simulink model "RailP_PRV"  (R2016b)
settings: configuration reference "CodeGenConfigSet" (kept outside this file)
values from neighbouring files (symbols this model uses):
  PRV_ClosePressureMin_C = Calibration.Parameter    [init_RailP_PRV.m]
  PRV_ctOpnMax_C = Calibration.Parameter    [init_RailP_PRV.m]
  PRV_dpRPGradOpn_CA0 = Calibration.Parameter    [init_RailP_PRV.m]
  PRV_dpRPGradOpn_CA1 = Calibration.Parameter    [init_RailP_PRV.m]
  PRV_nClsdMax_C = Calibration.Parameter    [init_RailP_PRV.m]
  PRV_nMinPresInc_C = Calibration.Parameter    [init_RailP_PRV.m]
  PRV_nOpnMin_C = Calibration.Parameter    [init_RailP_PRV.m]
  PRV_pAvrgRPTol_C = Calibration.Parameter    [init_RailP_PRV.m]
  PRV_tiCalcAvrgRP_C = Calibration.Parameter    [init_RailP_PRV.m]
  PRV_tiOpnMax_C = Calibration.Parameter    [init_RailP_PRV.m]
  PRV_tiWaitAvrgRP_C = Calibration.Parameter    [init_RailP_PRV.m]
  PRV_tiWaitNVld_C = Calibration.Parameter    [init_RailP_PRV.m]
  PRV_tiWaitPresInc_C = Calibration.Parameter    [init_RailP_PRV.m]
undefined symbols (not defined in the file or in its folder): PRV_State_conv, RailP_PRV_DT
settings Model: Creator=liutao  LastModifiedBy=shiliwei
settings ConfigSetRef: SourceLocation=Base Workspace

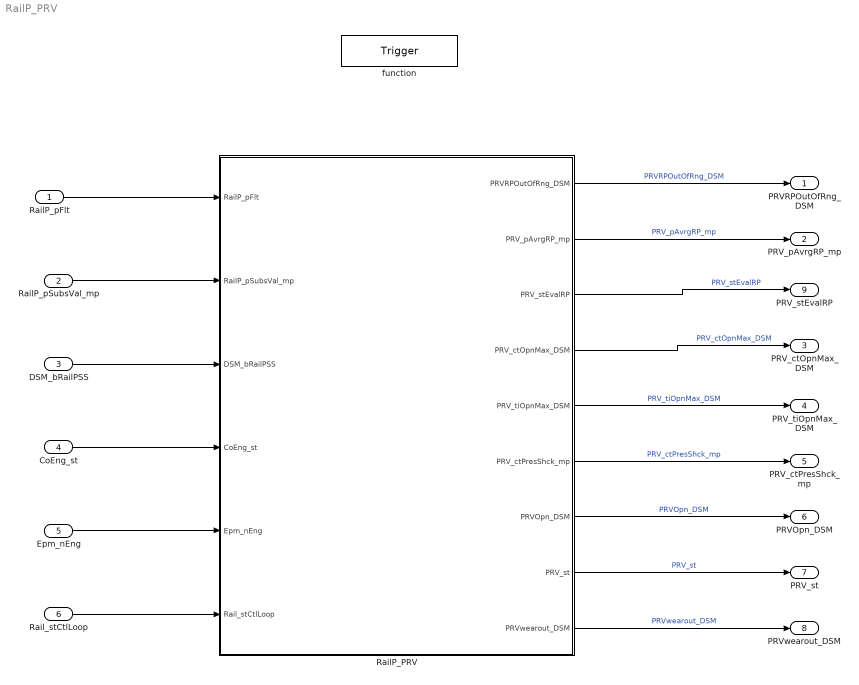
== system RailP_PRV ==
  RailP_pFlt : Inport  Tag=bar  Description=Maximum rail pressure of the last 10 sampling cycle  OutMin=0  OutMax=2500  OutDataTypeStr=RailPressure_bar
  RailP_pSubsVal_mp : Inport  Tag=bar  Description=Rail pressure substitution value in case of an error in pressure sensor  Port=2  OutMin=0  OutMax=2500  OutDataTypeStr=RailPressure_bar
  DSM_bRailPSS : Inport  Description=Status of FId_RailPSS  Port=3  OutMin=0  OutMax=1  OutDataTypeStr=boolean
  CoEng_st : Inport  Description=Engine coordinator state  Port=4  OutDataTypeStr=Enum: EngState_conv
  Epm_nEng : Inport  Tag=rpm  Description=Engine speed  Port=5  OutMin=0  OutMax=6000  OutDataTypeStr=EngSpeed_rpm
  Rail_stCtlLoop : Inport  Description=State of the rail pressure governor control  Port=6  OutDataTypeStr=Enum: RailCtl_State_conv
  function : TriggerPort  TriggerType=function-call  VariantControl=Variant
  RailP_PRV : Subsystem  TreatAsAtomicUnit=on
  PRVRPOutOfRng_DSM : Outport  Description=Averaged rail pressure is outside the expected tolerance range  OutMin=0  OutMax=1  OutDataTypeStr=boolean
  PRV_pAvrgRP_mp : Outport  Tag=bar  Description=|  Port=2  OutMin=0  OutMax=2000  OutDataTypeStr=RailPressure_bar
      | averaged rail pressure for detection of an opened
      | pressure relief valve by the rail pressure evaluation
  PRV_ctOpnMax_DSM : Outport  Description=Maximum number of opening cycles till wear out of PRV  Port=3  OutMin=0  OutMax=1  OutDataTypeStr=boolean
  PRV_tiOpnMax_DSM : Outport  Description=Maximum open time till wear out of PRV  Port=4  OutMin=0  OutMax=1  OutDataTypeStr=boolean
  PRV_ctPresShck_mp : Outport  Description=|  Port=5  OutMin=0  OutMax=6000  OutDataTypeStr=State_uint16
      | number of performed rail pressure shock cycles to
      | force the opening of the pressure relief valve
  PRVOpn_DSM : Outport  Description=PRV valve open state diagnostic  Port=6  OutMin=0  OutMax=1  OutDataTypeStr=boolean
  PRV_st : Outport  Description=state variable of the pressure relief valve  Port=7  OutDataTypeStr=Enum: PRV_State_conv
  PRVwearout_DSM : Outport  Description=PRV valve open counters or duration beyond setpoint value  Port=8  OutMin=0  OutMax=1  OutDataTypeStr=boolean
  PRV_stEvalRP : Outport  Description=state variable of the rail pressure evaluation for the recognition of the opening of the pressure relief valve  Port=9  OutDataTypeStr=Enum: PRV_EVALRPState_conv
  wires:
  RailP_PRV/1(PRVRPOutOfRng_DSM) -> PRVRPOutOfRng_DSM/1  "PRVRPOutOfRng_DSM"
  RailP_PRV/2(PRV_pAvrgRP_mp) -> PRV_pAvrgRP_mp/1  "PRV_pAvrgRP_mp"
  RailP_PRV/4(PRV_ctOpnMax_DSM) -> PRV_ctOpnMax_DSM/1  "PRV_ctOpnMax_DSM"
  RailP_PRV/5(PRV_tiOpnMax_DSM) -> PRV_tiOpnMax_DSM/1  "PRV_tiOpnMax_DSM"
  RailP_PRV/6(PRV_ctPresShck_mp) -> PRV_ctPresShck_mp/1  "PRV_ctPresShck_mp"
  RailP_PRV/7(PRVOpn_DSM) -> PRVOpn_DSM/1  "PRVOpn_DSM"
  RailP_PRV/8(PRV_st) -> PRV_st/1  "PRV_st"
  RailP_PRV/9(PRVwearout_DSM) -> PRVwearout_DSM/1  "PRVwearout_DSM"
  RailP_pFlt/1 -> RailP_PRV/1(RailP_pFlt)
  RailP_pSubsVal_mp/1 -> RailP_PRV/2(RailP_pSubsVal_mp)
  Rail_stCtlLoop/1 -> RailP_PRV/6(Rail_stCtlLoop)
  Epm_nEng/1 -> RailP_PRV/5(Epm_nEng)
  CoEng_st/1 -> RailP_PRV/4(CoEng_st)
  DSM_bRailPSS/1 -> RailP_PRV/3(DSM_bRailPSS)
  RailP_PRV/3("PRV_stEvalRP ") -> PRV_stEvalRP/1  "PRV_stEvalRP"

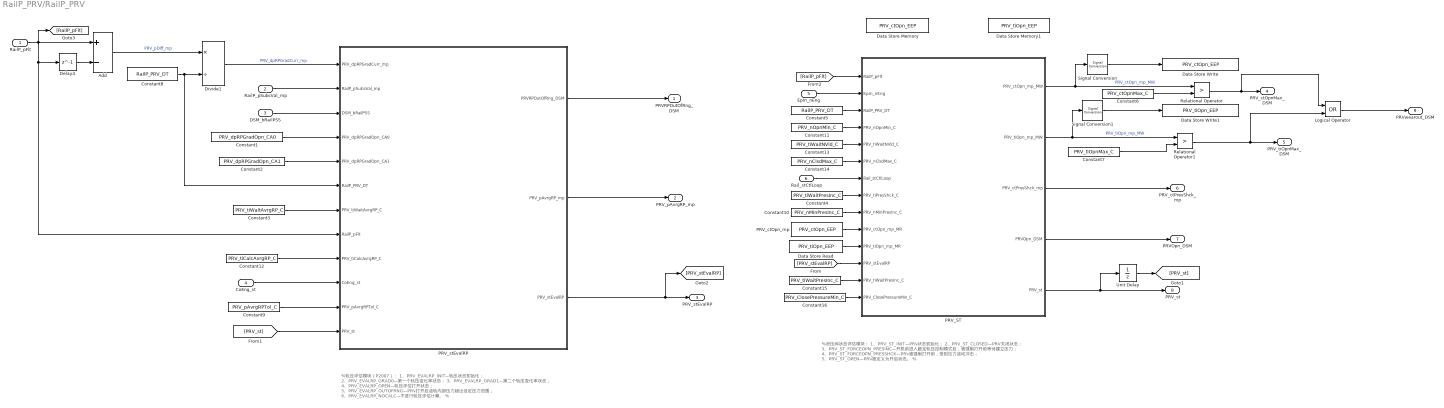
== system RailP_PRV/RailP_PRV ==
  note: %轨压评估模块（P2007）：
      | 1、PRV_EVALRP_INIT—轨压状态初始化；
      | 2、PRV_EVALRP_GRAD0—第一个轨压变化率状态；
      | 3、PRV_EVALRP_GRAD1—第二个轨压变化率状态；
      | 4、PRV_EVALRP_OPEN—轨压评估打开状态；
      | 5、PRV_EVALRP_OUTOFRNG—PRV打开后油轨内部压力超出设定压力范围；
      | 6、PRV_EVALRP_NOCALC—不进行轨压评估计算。
      | %
  note: %泄压阀状态评估模块：
      | 1、PRV_ST_INIT—PRV状态初始化；
      | 2、PRV_ST_CLOSED—PRV关闭状态；
      | 3、PRV_ST_FORCEOPN_PRESINC—开机前进入跛足轨压控制模式后，被强制打开前等待建立压力；
      | 4、PRV_ST_FORCEOPN_PRESSHCK—PRV被强制打开前，受到压力波动冲击；
      | 5、PRV_ST_OPEN—PRV被定义为开启状态。
      | %
  RailP_pFlt : Inport  Tag=mv  Description=Raw value of rail pressure
  RailP_pSubsVal_mp : Inport  Tag=mv  Description=Raw value of rail pressure  Port=2
  DSM_bRailPSS : Inport  Tag=mv  Description=Raw value of rail pressure  Port=3  OutMin=0  OutMax=1  OutDataTypeStr=boolean
  CoEng_st : Inport  Tag=mv  Description=Raw value of rail pressure  Port=4
  Epm_nEng : Inport  Tag=mv  Description=Raw value of rail pressure  Port=5
  Rail_stCtlLoop : Inport  Port=6
  Add : Sum  Inputs=+-  OutDataTypeStr=Inherit: Inherit via back propagation  InputSameDT=on
  Constant1 : Constant  Value=PRV_dpRPGradOpn_CA0
  Constant10 : Constant  Value=PRV_nMinPresInc_C
  Constant11 : Constant  Value=PRV_nOpnMin_C
  Constant12 : Constant  Value=PRV_tiCalcAvrgRP_C
  Constant13 : Constant  Value=PRV_tiWaitNVld_C
  Constant14 : Constant  Value=PRV_nClsdMax_C
  Constant15 : Constant  Value=PRV_tiWaitPresInc_C
  Constant16 : Constant  Value=PRV_ClosePressureMin_C
  Constant2 : Constant  Value=PRV_dpRPGradOpn_CA1
  Constant3 : Constant  Value=PRV_tiWaitAvrgRP_C
  Constant4 : Constant  Value=PRV_tiWaitPresInc_C
  Constant5 : Constant  Value=RailP_PRV_DT
  Constant6 : Constant  Value=PRV_ctOpnMax_C
  Constant7 : Constant  Value=PRV_tiOpnMax_C
  Constant8 : Constant  Value=RailP_PRV_DT
  Constant9 : Constant  Value=PRV_pAvrgRPTol_C
  Data Store Memory : DataStoreMemory  DataStoreName=PRV_ctOpn_EEP  ReadBeforeWriteMsg=warning  WriteAfterWriteMsg=warning  WriteAfterReadMsg=warning  ShowAdditionalParam=off
  Data Store Memory1 : DataStoreMemory  DataStoreName=PRV_tiOpn_EEP  ReadBeforeWriteMsg=warning  WriteAfterWriteMsg=warning  WriteAfterReadMsg=warning  ShowAdditionalParam=off  OutDataTypeStr=fixdt(0,32,10,0)
  Data Store Read : DataStoreRead  DataStoreName=PRV_tiOpn_EEP
  Data Store Write : DataStoreWrite  DataStoreName=PRV_ctOpn_EEP
  Data Store Write1 : DataStoreWrite  DataStoreName=PRV_tiOpn_EEP
  Delay4 : Delay  DelayLength=1  InitialCondition=0
  Divide1 : Product  Inputs=*/  OutDataTypeStr=Inherit: Inherit via back propagation  RndMeth=Round  SaturateOnIntegerOverflow=on
  Logical Operator : Logic  Operator=OR  AllPortsSameDT=off  OutDataTypeStr=boolean
  PRV_ST : Stateflow chart  TreatAsAtomicUnit=on
  PRV_ctOpn_mp : DataStoreRead  DataStoreName=PRV_ctOpn_EEP
  PRV_stEvalRP : Stateflow chart  TreatAsAtomicUnit=on
  Relational Operator : RelationalOperator  Operator=>  OutDataTypeStr=boolean  RndMeth=Simplest  InputSameDT=on
  Relational Operator1 : RelationalOperator  Operator=>  OutDataTypeStr=boolean  RndMeth=Simplest  InputSameDT=on
  Signal Conversion : SignalConversion  OverrideOpt=off
  Signal Conversion1 : SignalConversion  OverrideOpt=off
  Unit Delay : UnitDelay  InitialCondition=PRV_State_conv.PRV_ST_INIT  SampleTime=-1
  PRVRPOutOfRng_DSM : Outport  Tag=bar  Description=Maximum rail pressure of the last 10 sampling cycle  OutDataTypeStr=boolean
  PRV_pAvrgRP_mp : Outport  Tag=bar  Description=Maximum rail pressure of the last 10 sampling cycle  Port=2  OutMin=0  OutMax=2500
  "PRV_stEvalRP " : Outport  Tag=bar  Description=Maximum rail pressure of the last 10 sampling cycle  Port=3
  PRV_ctOpnMax_DSM : Outport  Tag=bar  Description=Maximum rail pressure of the last 10 sampling cycle  Port=4  OutMin=0  OutMax=1  OutDataTypeStr=boolean
  PRV_tiOpnMax_DSM : Outport  Tag=bar  Description=Maximum rail pressure of the last 10 sampling cycle  Port=5  OutMin=0  OutMax=1  OutDataTypeStr=boolean
  PRV_ctPresShck_mp : Outport  Tag=bar  Description=Maximum rail pressure of the last 10 sampling cycle  Port=6  OutMin=0  OutMax=2500
  PRVOpn_DSM : Outport  Tag=bar  Description=Maximum rail pressure of the last 10 sampling cycle  Port=7  OutMin=0  OutMax=1  OutDataTypeStr=boolean
  PRV_st : Outport  Tag=bar  Description=Maximum rail pressure of the last 10 sampling cycle  Port=8  OutDataTypeStr=Enum:PRV_State_conv
  PRVwearout_DSM : Outport  Tag=bar  Description=Maximum rail pressure of the last 10 sampling cycle  Port=9  OutMin=0  OutMax=1  OutDataTypeStr=boolean
  wires:
  Delay4/1 -> Add/2
  Add/1 -> Divide1/1  "PRV_pDiff_mp"
  Divide1/1 -> PRV_stEvalRP/1(PRV_dpRPGradCurr_mp)  "PRV_dpRPGradCurr_mp"
  RailP_pSubsVal_mp/1 -> PRV_stEvalRP/2(RailP_pSubsVal_mp)
  DSM_bRailPSS/1 -> PRV_stEvalRP/3(DSM_bRailPSS)
  Constant1/1 -> PRV_stEvalRP/4(PRV_dpRPGradOpn_CA0)
  Constant8/1 -> PRV_stEvalRP/6(RailP_PRV_DT), Divide1/2
  Constant3/1 -> PRV_stEvalRP/7(PRV_tiWaitAvrgRP_C)
  RailP_pFlt/1 -> [RailP_pFlt], Delay4/1, PRV_stEvalRP/8(RailP_pFlt), Add/1
  Constant12/1 -> PRV_stEvalRP/9(PRV_tiCalcAvrgRP_C)
  PRV_stEvalRP/1(PRVRPOutOfRng_DSM) -> PRVRPOutOfRng_DSM/1
  PRV_stEvalRP/2(PRV_pAvrgRP_mp) -> PRV_pAvrgRP_mp/1
  PRV_ST/1(PRV_ctOpn_mp_MW) -> Relational Operator/1, Signal Conversion/1  "PRV_ctOpn_mp_MW"
  PRV_ST/2(PRV_tiOpn_mp_MW) -> Relational Operator1/1, Signal Conversion1/1  "PRV_tiOpn_mp_MW"
  Constant5/1 -> PRV_ST/3(RailP_PRV_DT)
  Epm_nEng/1 -> PRV_ST/2(Epm_nEng)
  Rail_stCtlLoop/1 -> PRV_ST/7(Rail_stCtlLoop)
  Constant11/1 -> PRV_ST/4(PRV_nOpnMin_C)
  Constant13/1 -> PRV_ST/5(PRV_tiWaitNVld_C)
  Constant14/1 -> PRV_ST/6(PRV_nClsdMax_C)
  Constant4/1 -> PRV_ST/8(PRV_tiPresShck_C)
  Constant10/1 -> PRV_ST/9(PRV_nMinPresInc_C)
  PRV_ctOpn_mp/1 -> PRV_ST/10(PRV_ctOpn_mp_MR)
  Data Store Read/1 -> PRV_ST/11(PRV_tiOpn_mp_MR)
  PRV_ST/3(PRV_ctPresShck_mp) -> PRV_ctPresShck_mp/1
  Constant2/1 -> PRV_stEvalRP/5(PRV_dpRPGradOpn_CA1)
  CoEng_st/1 -> PRV_stEvalRP/10(CoEng_st)
  PRV_ST/4(PRVOpn_DSM) -> PRVOpn_DSM/1
  Signal Conversion/1 -> Data Store Write/1
  Signal Conversion1/1 -> Data Store Write1/1
  Relational Operator/1 -> Logical Operator/1, PRV_ctOpnMax_DSM/1
  Relational Operator1/1 -> Logical Operator/2, PRV_tiOpnMax_DSM/1
  Constant6/1 -> Relational Operator/2
  Constant7/1 -> Relational Operator1/2
  Constant9/1 -> PRV_stEvalRP/11(PRV_pAvrgRPTol_C)
  Constant15/1 -> PRV_ST/13(PRV_tiWaitPresInc_C)
  [PRV_stEvalRP] -> PRV_ST/12(PRV_stEvalRP)
  Unit Delay/1 -> [PRV_st]
  PRV_ST/5(PRV_st) -> Unit Delay/1, PRV_st/1
  [PRV_st] -> PRV_stEvalRP/12(PRV_st)
  PRV_stEvalRP/3(PRV_stEvalRP) -> [PRV_stEvalRP], "PRV_stEvalRP "/1
  Logical Operator/1 -> PRVwearout_DSM/1
  Constant16/1 -> PRV_ST/14(PRV_ClosePressureMin_C)
  [RailP_pFlt] -> PRV_ST/1(RailP_pFlt)

== stateflow chart RailP_PRV/PRV_stEvalRP ==
  state PRV_EVALRP_GRAD1
    en:
    PRV_stEvalRP=PRV_EVALRPState_conv.PRV_EVALRP_GRAD1 ;
    PRV_dpRPGrad1=PRV_dpRPGradCurr_mp;
    during:
    PRV_dpRPGrad1=PRV_dpRPGradCurr_mp;
  state PRV_EVALRP_GRAD0
    en:
    PRV_stEvalRP=PRV_EVALRPState_conv.PRV_EVALRP_GRAD0;
    PRV_dpRPGrad0=PRV_dpRPGradCurr_mp;
    during:
    PRV_dpRPGrad0=PRV_dpRPGradCurr_mp;
  state PRV_EVALRP_INIT
    entry:
    PRV_stEvalRP=PRV_EVALRPState_conv.PRV_EVALRP_INIT;
  state PRV_EVALRP_OPEN
    entry:
    PRV_stEvalRP=PRV_EVALRPState_conv.PRV_EVALRP_OPEN;
    m=0;
    n=0;
    x=0;
    flag=0;
    q=PRV_tiCalcAvrgRP_C/RailP_PRV_DT;
    during:
    m=m+RailP_PRV_DT;
    PRV_EVALRP_OPEN -> (junction 47) [order 1]
    (junction 47) -> (junction 48) [order 1] : [m>PRV_tiWaitAvrgRP_C]
    (junction 47) -> (junction 49) [order 2]
    (junction 48) -> (junction 50) : {n=n+RailP_PRV_DT;x=x+RailP_pFlt;}
    (junction 50) -> (junction 49)
    (junction 49) -> (junction 51)
    (junction 51) -> (junction 52) [order 1] : [n>PRV_tiCalcAvrgRP_C]
    (junction 51) -> (junction 54) [order 2]
    (junction 52) -> (junction 55) : {
        | PRV_pAvrgRP_mp=(x)/(q+1);
        | n=0;
        | x=0;
        | flag=1;
        | m=PRV_tiWaitAvrgRP_C;
        | }
    (junction 55) -> (junction 54)
    (junction 54) -> (junction 110)
    (junction 110) -> (junction 111) [order 1] : [((PRV_pAvrgRP_mp<=(RailP_pSubsVal_mp+PRV_pAvrgRPTol_C))&&(PRV_pAvrgRP_mp>=(RailP_pSubsVal_mp-PRV_pAvrgRPTol_C)))&&flag==1]
    (junction 110) -> (junction 112) [order 2]
    (junction 111) -> (junction 113) : {
        | flag=0;
        | }
    (junction 113) -> (junction 112)
    (junction 112) -> (junction 114)
  state PRV_EVALRP_OUTOFRNG
    entry:
    PRVRPOutOfRng_DSM=1;
    during:
    PRV_stEvalRP=PRV_EVALRPState_conv.PRV_EVALRP_OUTOFRNG;
  state PRV_EVALRP_NOCALC
    during:
    PRV_stEvalRP=PRV_EVALRPState_conv.PRV_EVALRP_NOCALC;
  (default) -> PRV_EVALRP_INIT
  PRV_EVALRP_GRAD0 -> PRV_EVALRP_GRAD1 [order 1] : [PRV_dpRPGrad0<PRV_dpRPGradOpn_CA0]
  PRV_EVALRP_INIT -> PRV_EVALRP_GRAD0 [order 2]
  PRV_EVALRP_GRAD1 -> PRV_EVALRP_GRAD0 [order 1] : [PRV_dpRPGrad1>PRV_dpRPGradOpn_CA1]
  PRV_EVALRP_INIT -> PRV_EVALRP_NOCALC [order 1] : [DSM_bRailPSS==0]
  PRV_EVALRP_NOCALC -> PRV_EVALRP_GRAD0 : [DSM_bRailPSS==1]
  PRV_EVALRP_GRAD0 -> PRV_EVALRP_NOCALC [order 2] : [DSM_bRailPSS==0]
  PRV_EVALRP_OUTOFRNG -> PRV_EVALRP_GRAD0 [order 1] : [PRV_st==PRV_State_conv.PRV_ST_CLOSED]{PRVRPOutOfRng_DSM=0;}
  PRV_EVALRP_OPEN -> PRV_EVALRP_GRAD0 [order 3] : [PRV_st==PRV_State_conv.PRV_ST_CLOSED]
  PRV_EVALRP_GRAD1 -> PRV_EVALRP_NOCALC [order 3] : [DSM_bRailPSS==0]
  PRV_EVALRP_GRAD1 -> PRV_EVALRP_OPEN [order 2] : [PRV_dpRPGrad1<PRV_dpRPGradOpn_CA1]
  PRV_EVALRP_OPEN -> PRV_EVALRP_OUTOFRNG [order 1] : [((PRV_pAvrgRP_mp>=(RailP_pSubsVal_mp+PRV_pAvrgRPTol_C))||...
      | (PRV_pAvrgRP_mp<=(RailP_pSubsVal_mp-PRV_pAvrgRPTol_C)))&&flag==1]
  PRV_EVALRP_OUTOFRNG -> PRV_EVALRP_NOCALC [order 2] : [DSM_bRailPSS==0]
  PRV_EVALRP_OPEN -> PRV_EVALRP_NOCALC [order 2] : [DSM_bRailPSS==0]
  data: n local uint16 size=1 =0; x local uint32 size=1 =0; q local uint16 size=1 =0; PRV_dpRPGradCurr_mp input; RailP_pSubsVal_mp input; DSM_bRailPSS input; PRVRPOutOfRng_DSM output; PRV_dpRPGradOpn_CA0 input; PRV_dpRPGradOpn_CA1 input; RailP_PRV_DT input; PRV_tiWaitAvrgRP_C input; RailP_pFlt input; PRV_tiCalcAvrgRP_C input; PRV_pAvrgRP_mp output RailPressure_bar; PRV_stEvalRP output Enum: PRV_EVALRPState_conv =PRV_EVALRPState_conv.PRV_EVALRP_INIT; CoEng_st input; PRV_pAvrgRPTol_C input; PRV_st input; flag local uint8 size=1 =0; PRV_dpRPGrad0 local RailPressure_bar_ms size=1 =0; PRV_dpRPGrad1 local RailPressure_bar_ms size=1 =0; m local uint16 size=1 =0

== stateflow chart RailP_PRV/PRV_ST ==
  state PRV_ST_CLOSED
    entry:
    PRV_st=PRV_State_conv.PRV_ST_CLOSED;
    PRVOpn_DSM=0;
    during:
    PRV_ctPresShck_mp=0;
  state PRV_ST_FORCEOPN_PRESSHCK
    entry:
    PRV_ctPresShck_mp=PRV_ctPresShck_mp+1;
    b=0;
    PRV_st=PRV_State_conv.PRV_ST_FORCEOPN_PRESSHCK;
    during:
    b=b+RailP_PRV_DT;%模块采样时间10ms
  state PRV_ST_FORCEOPN_PRESINC
    entry:
    c=0;
    PRV_st=PRV_State_conv.PRV_ST_FORCEOPN_PRESINC;
    during:
    c=c+RailP_PRV_DT;%模块采样时间10ms
  state PRV_ST_INIT
    entry:
    PRV_st=PRV_State_conv.PRV_ST_INIT;
    PRVOpn_DSM=0;
    a=0;
    PRV_ctOpn_mp_MW=PRV_ctOpn_mp_MR;
    PRV_tiOpn_mp_MW=PRV_tiOpn_mp_MR;
    during:
    a=a+RailP_PRV_DT;%模块采样时间10ms
  state PRV_ST_OPEN
    entry:
    PRV_ctOpn_mp_MW=PRV_ctOpn_mp_MW+1;%开启次数
    PRV_st=PRV_State_conv.PRV_ST_OPEN;
    PRVOpn_DSM=1;
    PRV_ctPresShck_mp=0;
    during:
    PRV_tiOpn_mp_MW=PRV_tiOpn_mp_MW+RailP_PRV_DT;%开启累计时间写入E2
  PRV_ST_FORCEOPN_PRESSHCK -> PRV_ST_CLOSED [order 2] : [Epm_nEng<PRV_nClsdMax_C]
  PRV_ST_INIT -> PRV_ST_CLOSED [order 1] : [(Epm_nEng < PRV_nOpnMin_C)&&(a>=PRV_tiWaitNVld_C)]
  PRV_ST_FORCEOPN_PRESINC -> PRV_ST_CLOSED [order 2] : [Epm_nEng<PRV_nClsdMax_C]
  PRV_ST_CLOSED -> PRV_ST_FORCEOPN_PRESINC [order 2] : [(Epm_nEng>PRV_nClsdMax_C)&&(Rail_stCtlLoop ==RailCtl_State_conv.RAIL_LIMP_NOCTL || Rail_stCtlLoop == RailCtl_State_conv.RAIL_LIMP_OPENCTL)]
  PRV_ST_OPEN -> PRV_ST_CLOSED : [(Epm_nEng<PRV_nClsdMax_C)||(RailP_pFlt<PRV_ClosePressureMin_C)]
  PRV_ST_CLOSED -> PRV_ST_OPEN [order 1] : [(Epm_nEng>PRV_nClsdMax_C )&&(PRV_stEvalRP==PRV_EVALRPState_conv.PRV_EVALRP_OPEN)]
  PRV_ST_FORCEOPN_PRESSHCK -> PRV_ST_FORCEOPN_PRESINC [order 1] : [b>PRV_tiPresShck_C]
  PRV_ST_FORCEOPN_PRESINC -> PRV_ST_FORCEOPN_PRESSHCK [order 1] : [(c>PRV_tiWaitPresInc_C)&&(Epm_nEng>PRV_nMinPresInc_C)]
  PRV_ST_FORCEOPN_PRESSHCK -> PRV_ST_OPEN [order 3] : [PRV_stEvalRP==PRV_EVALRPState_conv.PRV_EVALRP_OPEN]
  PRV_ST_FORCEOPN_PRESINC -> PRV_ST_OPEN [order 3] : [PRV_ctPresShck_mp>0&&((PRV_stEvalRP==PRV_EVALRPState_conv.PRV_EVALRP_NOCALC)||(PRV_stEvalRP==PRV_EVALRPState_conv.PRV_EVALRP_OPEN))]
  (default) -> PRV_ST_INIT
  PRV_ST_INIT -> PRV_ST_OPEN [order 2] : [(Epm_nEng > PRV_nOpnMin_C)]
  data: RailP_pFlt input; Epm_nEng input; RailP_PRV_DT input; PRV_nOpnMin_C input; PRV_tiWaitNVld_C input; PRV_nClsdMax_C input; Rail_stCtlLoop input; PRV_tiPresShck_C input; PRV_nMinPresInc_C input; PRV_ctOpn_mp_MR input State_uint8; PRV_tiOpn_mp_MR input EngTime_ms; PRV_ctOpn_mp_MW output uint8; PRV_tiOpn_mp_MW output EngTime_ms; PRV_stEvalRP input; PRV_ctPresShck_mp output; PRVOpn_DSM output boolean; PRV_st output; PRV_tiWaitPresInc_C input; a local uint32 size=1; b local uint32 size=1; c local uint32 size=1; PRV_ClosePressureMin_C input
